simulink model "Exercitiul3"  (R2016a)
settings: Solver=VariableStepDiscrete  StartTime=0.0  StopTime=480  RelTol=1e-3
undefined symbols (not defined in the file): m, n
settings Model: Creator=Cristina  LastModifiedBy=Cristina

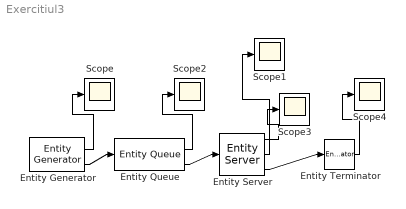
== system Exercitiul3 ==
  Entity Generator : EntityGenerator  OutputPortMessageModes=n,m  TimeSource=MATLAB action  IntergenerationTimeAction=dt = 12 + 12 * rand;  NumberEntitiesDeparted=on  EntityType=Structured  EntityTypeName=Entity
      settings: OutputPortMap=o0,o3
  Entity Queue : EntityQueue  InputPortMessageModes=m  OutputPortMessageModes=n,m  AverageWait=on
      settings: OutputPortMap=o2,o5
  Entity Server : EntityServer  InputPortMessageModes=m  OutputPortMessageModes=n,n,m  Capacity=2  ServiceTimeSource=MATLAB action  ServiceTimeAction=dt = 28 + 8 * rand;  AverageWait=on  Utilization=on
      settings: OutputPortMap=o4,o5,o9
  Entity Terminator : EntityTerminator  InputPortMessageModes=m  NumberEntitiesArrived=on
      settings: OutputPortMap=o0
  Scope{,1..4} (5 alike) : Scope
  wires:
  Entity Server/3 -> Entity Terminator/1
  Entity Generator/2 -> Entity Queue/1
  Entity Generator/1 -> Scope/1
  Entity Queue/2 -> Entity Server/1
  Entity Queue/1 -> Scope2/1
  Entity Server/1 -> Scope3/1
  Entity Server/2 -> Scope1/1
  Entity Terminator/1 -> Scope4/1
